simulink model "Piccolo_Induction_Motor"  (R2022b)
settings: Solver=FixedStepAuto  StartTime=0.0  StopTime=Inf  RelTol=1e-3  EnableMultiTasking=on
PostLoadFcn:
  | ,try, rti_mdl_postloadfcn(bdroot, 'UpdateModel', 320, 'rti1104'); catch, disp(lasterr); end,
undefined symbols (not defined in the file or in its folder): Km
libraries: Piccolo_Library x4, c2802xlib x1
settings Model: ExtModeTrigDuration=8  Creator=sb35user  LastModifiedBy=carls
settings SolverCC: ZeroCrossAlgorithm=Non-adaptive  AlgebraicLoopSolver=TrustRegion  AutoInsertRateTranBlk=on
settings DataIOCC: LimitDataPoints=on  SaveFormat=Array  SignalLoggingSaveFormat=ModelDataLogs  ReturnWorkspaceOutputs=off
settings OptimizationCC: BlockReduction=off  DefaultUnderspecifiedDataType=single  EnhancedBackFolding=on  PassReuseOutputArgsAs=Individual arguments  ExpressionDepthLimit=2147483647  InitFltsAndDblsToZero=on  MaxStackSize=1024  OptimizeBlockOrder=speed  DifferentSizesBufferReuse=on  OptimizationCustomize=off  DenormalBehavior=FlushToZero  EfficientTunableParamExpr=on
settings DebuggingCC: UnderspecifiedInitializationDetection=Classic  MergeDetectMultiDrivingBlocksExec=none  SolverPrmCheckMsg=warning  ParameterTunabilityLossMsg=error  FcnCallInpInsideContextMsg=warning  UnconnectedInputMsg=warning  UnconnectedOutputMsg=warning  UnconnectedLineMsg=warning  StateNameClashWarn=warning  SFUnexpectedBacktrackingDiag=warning  SFNoUnconditionalDefaultTransitionDiag=warning  SFExecutionAtInitializationDiag=none  SFMachineParentedDataDiag=warning  ArithmeticOperatorsInVariantConditions=warning
settings HardwareCC: ProdBitPerChar=16  ProdBitPerInt=16  ProdBitPerPointer=32  ProdBitPerSizeT=32  ProdBitPerPtrDiffT=32  ProdLargestAtomicInteger=Integer  ProdLargestAtomicFloat=None  ProdWordSize=16  ProdLongLongMode=on  ProdHWDeviceType=Texas Instruments->C2000  TargetIntDivRoundTo=Zero  TargetEndianess=BigEndian
settings ModelReferenceCC: PropagateSignalLabelsOutOfModel=off
settings SFSimCC: MATLABDynamicMemAlloc=off
settings RTWCC: Description=Embedded Coder  SystemTargetFile=ert.tlc  HardwareBoard=TI Piccolo F28069M LaunchPad  TLCOptions=-aInlineSetEventsForThisBaseRateFcn=TLC_FALSE -aSuppressMultiTaskScheduler=TLC_FALSE -aRateBasedStepFcn=1  TemplateMakefile=ert_default_tmf  Toolchain=Texas Instruments Code Composer Studio (C2000)
settings CodeAppCC: ForceParamTrailComments=on  IgnoreCustomStorageClasses=off  OperatorAnnotations=on  SimulinkDataObjDesc=on  SFDataObjDesc=on  InsertBlockDesc=on
settings ERTTargetCC: CodeReplacementLibrary=TI C28x  SupportContinuousTime=on  ExtModeTransport=4  ExtModeStaticAlloc=on  ExtModeAutomaticAllocSize=off  ExtModeMexFile=ext_xcp  ExtModeIntrfLevel=Level2 - Open
settings ConfigComp: CovMetricSettings=dw  CovSaveCumulativeToWorkspaceVar=on  CovSaveSingleToWorkspaceVar=on

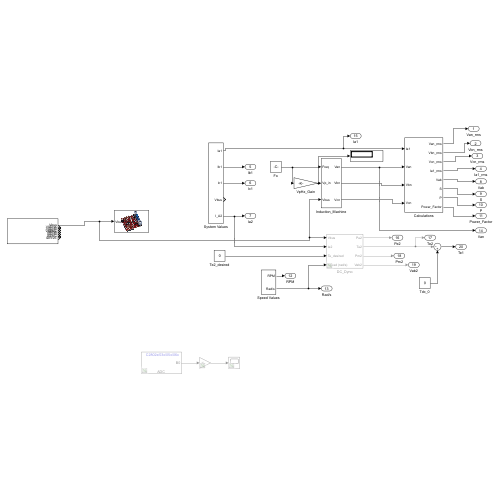
[thumbnail: Simulink's stored preview of the top-level diagram]
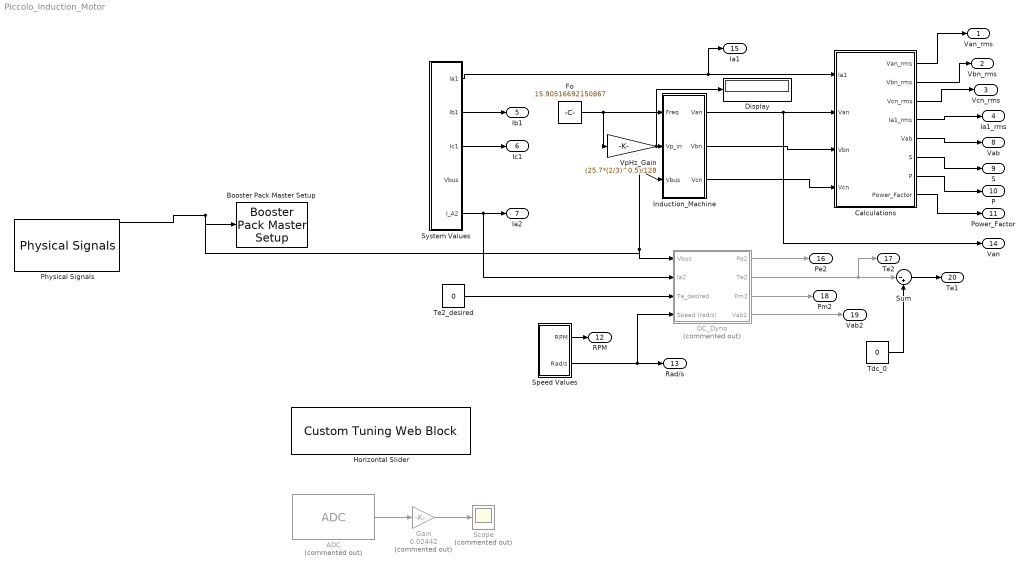
== system Piccolo_Induction_Motor ==
  ADC : c2802xlib/ADC  Commented=on  blkParamProc=C2000  ADCModule=1  samplingMode=Single sample mode  ADCResolution=12-bit (Single-ended input)  useSOC1=SOC0  useSOC2=SOC0_SOC1  SOCAcquisitionWindow=8  SOCTriggerSource=Software  SOCInterruptTrigger=No ADCINT  Ts=50e-6  dType=uint16  postInterrupt=off  interruptSel=ADCINT1  ADCINTContinuous=off  endma=off  chdma=1  conv1=ADCINB0  conv2=ADCINA0 and ADCINB0  conv1_Type4=ADCIN0  conv2_Type4=ADCIN0 and ADCIN1
      settings: LibrarySourceBlock=c2806xlib/ADC
  Booster Pack Master Setup : Piccolo_Library/Booster Pack Master Setup  SystemSampleTime=-1  VariantActivationTime=update diagram  Latency=0  AutoFrameSizeCalculation=off
      settings: SourceProductName=Piccolo Motor Control
  Calculations : Subsystem
  DC_Dyno : Subsystem  Commented=on
  Display : Display
  Fo : Constant  Value=15.90516692150867
  Gain : Gain  Commented=on  Gain=0.02442
  Horizontal Slider : CustomTuningWebBlock  LabelPosition=Hide  ShowInitialText=on  Configuration="{\"components\":[{\"name\":\"LinearScaleComponent\",\"settings\":{\"bounds\":{\"max\":60,\"min\":10,\"tickInterval\":\"auto\"},\"internalTickHeightScaleFactor\":0.5,\"labelColor\":[255,255,200],\"labelFont\":{\"font\":\"Arial\",\"fontSize\":12},\"labelOffset\":0.05,\"labelTransparency\":1,\"needleImage\":{\"size\":[596,842],\"src\":\"data:image\\/svg+xml;base64,PD94bWwgdmVyc2lvbj0iMS4wIiBlbmNvZGluZz0idXRmLTgiPz4NCjwhLS0gR2VuZXJhdG9yOiBBZG9iZSBJbGx1c3RyYXRvciAyNS4wLjAsIFNWRyBFeHBvcnQgUGx1Zy1JbiAuIFNWRyBWZXJzaW9uOiA2LjAwIEJ1aWxkIDApICAtLT4NCjxzdmcgdmVyc2lvbj0iMS4xIg0KCSBpZD0ic3ZnOCIgeG1sbnM6Y2M9Imh0dHA6Ly9jcmVhdGl2ZWNvbW1vbnMub3JnL25zIyIgeG1sbnM6ZGM9Imh0dHA6Ly9wdXJsLm9yZy9kYy9lbGVtZW50cy8xLjEvIiB4bWxuczppbmtzY2FwZT0iaHR0cDovL3d3dy5pbmtzY2FwZS5vcmcvbmFtZXNw ...(+2420 chars)\",\"srcOrientation\":\"Right\"},\"needleOffset\":[-0.8044596912521441,-0.0642123287671233],\"needleSize\":{\"height\":0.4337797619047619,\"width\":0.07668067226890757},\"position\":[0.2829861111111111,0.04398634453781513,0.9196428571428571,0.6088789682539683],\"referencePoint\":\"auto\",\"scaleColors\":[],\"scaleColorsSize\":0.2,\"scaleDirection\":\"LR\",\"showLabels\":1,\"showMinorTicks\":0,\"showSpanLine\":1,\"showTicks\":1,\"tickColor\":[252,252,197],\"tickTransparency\":1,\"valueBarColor\":[0,114,189],\"valueBarOffset\":-0.27,\"valueBarSize\":0.1,\"valueBarTransparency\":1}},{\"name\":\"BackgroundImageComponent\",\"settings\":{\"image\":{\"size\":[380,101],\"src\":\"data:image\\/svg+xml;base64,PHN2ZyB4bWxucz0iaHR0cDovL3d3dy53My5vcmcvMjAwMC9zdmciIHhtbG5zOnhsaW5rPSJodHRwOi8vd3d3LnczLm9yZy8xOTk5L3hsaW5rIiB2aWV3Qm94PSIwIDAgMzgwIDEwMSI+PGRlZnM+PHN0eWxlPi5jbHMtMXtmaWxsOiMwMDJiNDI7fS5jbHMtMntmaWxsOiM0MjcwODI7fS5jbHMtM3tmaWxsOnVybCgjcmFkaWFsLWdyYWRpZW50KTt9LmNscy00e2ZpbGw6I2M4YzhjODtzdHJva2U6IzAwMDt9PC9zdHlsZT48cmFkaWFsR3JhZGllbnQgaWQ9InJhZGlhbC1ncmFkaWVudCIgY3g9IjE5MCIgY3k9IjUwLjUiIHI9IjI2OS4yMSIgZ3JhZGllbnRVbml0cz0idXNlclNwYWNlT25Vc2UiPjxzdG9wIG9mZnNldD0iMC4wMSIgc3RvcC1jb2xvcj0iIzNlNGY1OCIvPjxzdG9wIG9mZnNldD0iMC4wNiIgc3RvcC1jb2xvcj0iIzQ0NTc2MSIvPjxzdG9wIG9mZnNldD0iMC4xNSIgc3RvcC1jb2xvcj0iIzU1NmE3NiIvPjxzdG9wIG9mZnNldD0iMC4yNSIgc3RvcC1jb2xvcj0iIzZkODg5NSIvPjxzdG9wIG9mZnNldD0iMC4zOCIgc3RvcC1jb2xvcj0iIzhmYjJjMyIvPjxzdG9wIG9mZnNldD0iMC41MiIgc3RvcC1jb2xvcj0iI2I2ZTRmYSIvPjxzdG9wIG9mZnNldD0iMSIgc3RvcC1jb2xvcj0iIzE1NDY1NyIvPjwvcmFkaWFsR3JhZGllbnQ+PC9kZWZzPjxnIGlkPSJmcmFtZSI+PGcgaWQ9IkxheWVyXzIiIGRhdGEtbmFtZT0iTGF5ZXIgMiI+PGcgaWQ9IkxheWVyXzEtMiIgZGF0YS1uYW1lPSJMYXllciAxLTIiPjxyZWN0IGlkPSJyZWN0MTAzNiIgY2xhc3M9ImNscy0xIiB4PSIxMSIgeT0iMTEiIHdpZHRoPSIzNTgiIGhlaWdodD0iNzkiLz48cGF0aCBpZD0icGF0aDEwMzgiIGNsYXNzPSJjbHMtMiIgZD0iTTgsOFY5M0gzNzJWOFpNMzY5LDkwSDExVjExSDM2OVoiLz48cGF0aCBpZD0icGF0aDEwNDAiIGNsYXNzPSJjbHMtMyIgZD0iTTAsMFYxMDFIMzgwVjBaTTM3Miw5M0g4VjhIMzcyWiIvPjwvZz48L2c+PC9nPjxnIGlkPSJ0cmFjayI+PHBhdGggaWQ9InJlY3QxNjExIiBjbGFzcz0iY2xzLTQiIGQ9Ik0zMy4zNywyNi41OUgzNDYuNjNjNCwwLDcuMjUsMi42LDcuMjUsNS44MWgwYzAsMy4yMS0zLjI1LDUuODItNy4yNSw1LjgySDMzLjM3Yy00LDAtNy4yNS0yLjYxLTcuMjUtNS44MmgwQzI2LjEyLDI5LjE5LDI5LjM3LDI2LjU5LDMzLjM3LDI2LjU5WiIvPjwvZz48L3N2Zz4=\",\"srcOrientation\":\"horizontal\"},\"position\":[0,0,1,1],\"scaleMode\":\"0\"}},{\"name\":\"ForegroundImageComponent\",\"settings\":{\"image\":{\"size\":[0,0],\"src\":\"default\",\"srcOrientation\":[]},\"isForeground\":1,\"position\":[0,0,1,1],\"scaleMode\":\"0\"}}],\"settings\":{\"BindingType\":\"param\",\"aspectRatio\":3.7777777777777777,\"backgroundColor\":[0,0,0,\"1\"],\"backgroundOffset\":0,\"backgroundOpacity\":1,\"fixedAspectRatio\":\"on\",\"foregroundColor\":[252,252,196],\"orientation\":\"horizontal\",\"showBackgroundColor\":false,\"value\":0,\"version\":\"R2022b\"},\"type\":\"LinearGauge\"}"
  Induction_Machine : Subsystem
  Physical Signals : Piccolo_Library/Physical Signals  Pack=1
      settings: SourceProductName=Piccolo Motor Control
  Scope : Scope  Commented=on
  Speed Values : Subsystem
  Sum : Sum  Inputs=|-+
  System Values : Subsystem
  Tdc_0 : Constant  Value=0
  Te2_desired : Constant  Value=0
  VpHz_Gain : Gain  Gain=(25.7*(2/3)^0.5)/128
  Van_rms : Outport
  Vbn_rms : Outport  Port=2
  Vcn_rms : Outport  Port=3
  Ia1_rms : Outport  Port=4
  Ib1 : Outport  Port=5
  Ic1 : Outport  Port=6
  Ia2 : Outport  Port=7
  Vab : Outport  Port=8
  S : Outport  Port=9
  P : Outport  Port=10
  Power_Factor : Outport  Port=11
  RPM : Outport  Port=12
  Rad/s : Outport  Port=13
  Van : Outport  Port=14
  Ia1 : Outport  Port=15
  Pe2 : Outport  Port=16
  Te2 : Outport  Port=17
  Pm2 : Outport  Port=18
  Vab2 : Outport  Port=19
  Te1 : Outport  Port=20
  wires:
  System Values/2(Ib1) -> Ib1/1
  System Values/3(Ic1) -> Ic1/1
  Fo/1 -> Induction_Machine/1(Freq), VpHz_Gain/1
  System Values/5(I_A2) -> Ia2/1, DC_Dyno/2(Ia2)
  Induction_Machine/3(Vcn) -> Calculations/4(Vcn)
  System Values/1(Ia1) -> Calculations/1(Ia1), Ia1/1
  Induction_Machine/1(Van) -> Calculations/2(Van), Van/1
  Induction_Machine/2(Vbn) -> Calculations/3(Vbn)
  Calculations/1(Van_rms) -> Van_rms/1
  Calculations/2(Vbn_rms) -> Vbn_rms/1
  Calculations/3(Vcn_rms) -> Vcn_rms/1
  Calculations/4(Ia1_rms) -> Ia1_rms/1
  Calculations/5(Vab) -> Vab/1
  Calculations/6(S) -> S/1
  Calculations/7(P) -> P/1
  Calculations/8(Power_Factor) -> Power_Factor/1
  Speed Values/1(RPM) -> RPM/1
  Speed Values/2(Rad/s) -> Rad/s/1, DC_Dyno/4(Speed (rad/s))
  Te2_desired/1 -> DC_Dyno/3(Te_desired)
  DC_Dyno/1(Pe2) -> Pe2/1
  DC_Dyno/3(Pm2) -> Pm2/1
  DC_Dyno/4(Vab2) -> Vab2/1
  DC_Dyno/2(Te2) -> Sum/1, Te2/1
  Tdc_0/1 -> Sum/2
  Sum/1 -> Te1/1
  Physical Signals/1 -> Induction_Machine/3(Vbus), DC_Dyno/1(Vbus), Booster Pack Master Setup/1
  Gain/1 -> Scope/1
  ADC/1 -> Gain/1
  VpHz_Gain/1 -> Display/1, Induction_Machine/2(Vp_in)

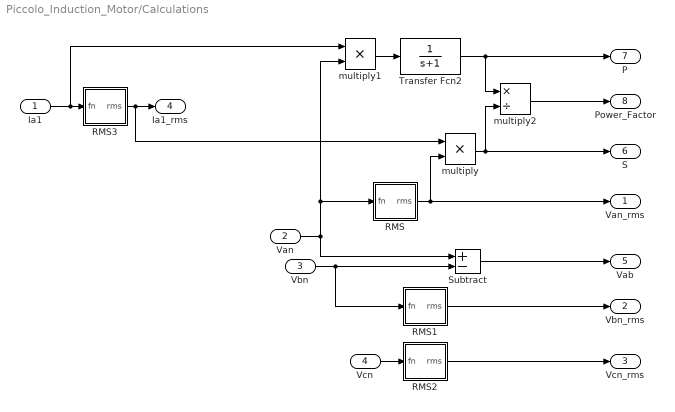
== system Piccolo_Induction_Motor/Calculations ==
  Ia1 : Inport
  Van : Inport  Port=2
  Vbn : Inport  Port=3
  Vcn : Inport  Port=4
  RMS : Subsystem
  RMS1 : Subsystem
  RMS2 : Subsystem
  RMS3 : Subsystem
  Subtract : Sum  Inputs=+-
  Transfer Fcn2 : TransferFcn  Denominator=[1 1]
  multiply : Product  Inputs=**
  multiply1 : Product  Inputs=**
  multiply2 : Product  Inputs=*/
  Van_rms : Outport
  Vbn_rms : Outport  Port=2
  Vcn_rms : Outport  Port=3
  Ia1_rms : Outport  Port=4
  Vab : Outport  Port=5
  S : Outport  Port=6
  P : Outport  Port=7
  Power_Factor : Outport  Port=8
  wires:
  Subtract/1 -> Vab/1
  Van/1 -> multiply1/2, RMS/1(fn), Subtract/1
  Vbn/1 -> RMS1/1(fn), Subtract/2
  RMS/1(rms) -> Van_rms/1, multiply/2
  RMS1/1(rms) -> Vbn_rms/1
  RMS2/1(rms) -> Vcn_rms/1
  Ia1/1 -> multiply1/1, RMS3/1(fn)
  RMS3/1(rms) -> Ia1_rms/1, multiply/1
  multiply/1 -> S/1, multiply2/2
  Transfer Fcn2/1 -> P/1, multiply2/1
  multiply1/1 -> Transfer Fcn2/1
  multiply2/1 -> Power_Factor/1
  Vcn/1 -> RMS2/1(fn)

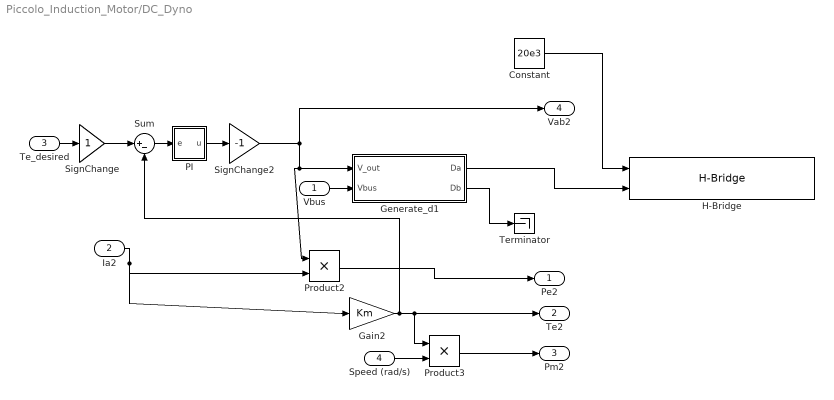
== system Piccolo_Induction_Motor/DC_Dyno ==
  Vbus : Inport
  Ia2 : Inport  Port=2
  Te_desired : Inport  Port=3
  Speed (rad/s) : Inport  Port=4
  Constant : Constant  Value=20e3
  Gain2 : Gain  Gain=Km
  Generate_d1 : Subsystem
  H-Bridge : Piccolo_Library/H-Bridge  Pack=1  Prescale=8
      settings: SourceProductName=Piccolo Motor Control
  PI : Subsystem
  Product2 : Product  RndMeth=Zero
  Product3 : Product  RndMeth=Zero
  SignChange : Gain
  SignChange2 : Gain  Gain=-1
  Sum : Sum  Inputs=|+-
  Terminator : Terminator
  Pe2 : Outport
  Te2 : Outport  Port=2
  Pm2 : Outport  Port=3
  Vab2 : Outport  Port=4
  wires:
  PI/1(u) -> SignChange2/1
  Generate_d1/1(Da) -> H-Bridge/2
  Generate_d1/2(Db) -> Terminator/1
  Product2/1 -> Pe2/1
  Product3/1 -> Pm2/1
  Sum/1 -> PI/1(e)
  Gain2/1 -> Sum/2, Te2/1, Product3/1
  Vbus/1 -> Generate_d1/2(Vbus)
  Ia2/1 -> Product2/2, Gain2/1
  Speed (rad/s)/1 -> Product3/2
  Te_desired/1 -> SignChange/1
  SignChange/1 -> Sum/1
  SignChange2/1 -> Product2/1, Generate_d1/1(V_out), Vab2/1
  Constant/1 -> H-Bridge/1

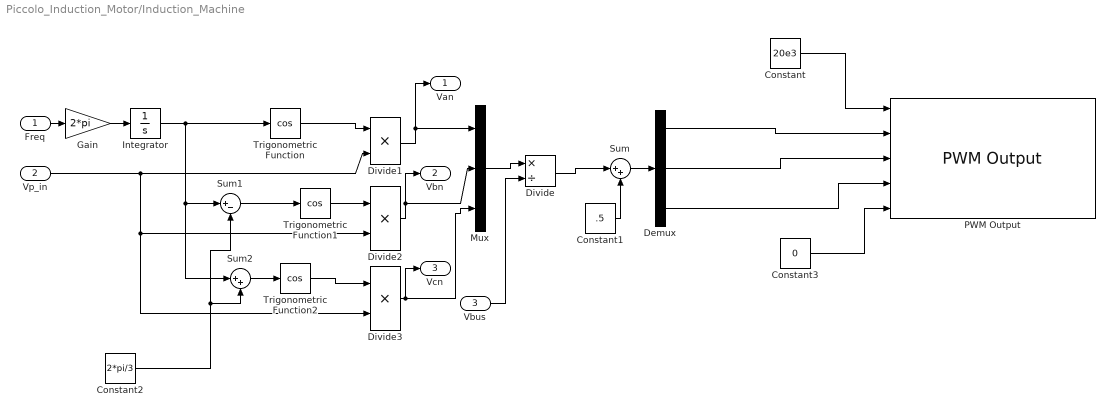
== system Piccolo_Induction_Motor/Induction_Machine ==
  Freq : Inport
  Vp_in : Inport  Port=2
  Vbus : Inport  Port=3
  Constant : Constant  Value=20e3
  Constant1 : Constant  Value=.5
  Constant2 : Constant  Value=2*pi/3
  Constant3 : Constant  Value=0
  Demux : Demux  Outputs=3
  Divide : Product  Inputs=*/
  Divide1 : Product  Inputs=**
  Divide2 : Product  Inputs=**
  Divide3 : Product  Inputs=**
  Gain : Gain  Gain=2*pi
  Integrator : Integrator
  Mux : Mux  Inputs=3
  PWM Output : Piccolo_Library/PWM Output  Pack=1  Prescale=1
      settings: SourceProductName=Piccolo Motor Control
  Sum : Sum  Inputs=|++
  Sum1 : Sum  Inputs=|+-
  Sum2 : Sum  Inputs=|++
  Trigonometric Function : Trigonometry  Operator=cos
  Trigonometric Function1 : Trigonometry  Operator=cos
  Trigonometric Function2 : Trigonometry  Operator=cos
  Van : Outport
  Vbn : Outport  Port=2
  Vcn : Outport  Port=3
  wires:
  Constant1/1 -> Sum/2
  Sum/1 -> Demux/1
  Mux/1 -> Divide/1
  Divide/1 -> Sum/1
  Vbus/1 -> Divide/2
  Gain/1 -> Integrator/1
  Freq/1 -> Gain/1
  Integrator/1 -> Trigonometric Function/1, Sum2/1, Sum1/1
  Trigonometric Function/1 -> Divide1/1
  Vp_in/1 -> Divide1/2, Divide2/2, Divide3/2
  Divide1/1 -> Mux/1, Van/1
  Sum1/1 -> Trigonometric Function1/1
  Divide2/1 -> Mux/2, Vbn/1
  Trigonometric Function1/1 -> Divide2/1
  Constant2/1 -> Sum1/2, Sum2/2
  Sum2/1 -> Trigonometric Function2/1
  Trigonometric Function2/1 -> Divide3/1
  Divide3/1 -> Mux/3, Vcn/1
  Demux/1 -> PWM Output/2
  Demux/2 -> PWM Output/3
  Demux/3 -> PWM Output/4
  Constant/1 -> PWM Output/1
  Constant3/1 -> PWM Output/5

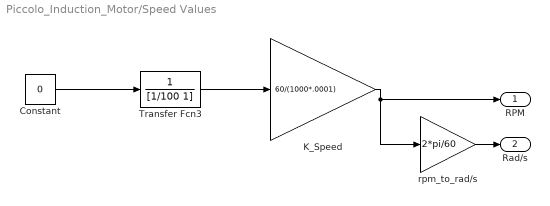
== system Piccolo_Induction_Motor/Speed Values ==
  Constant : Constant  Value=0
  K_Speed : Gain  Gain=60/(1000*.0001)
  Transfer Fcn3 : TransferFcn  Denominator=[1/100 1]
  rpm_to_rad/s : Gain  Gain=2*pi/60
  RPM : Outport
  Rad/s : Outport  Port=2
  wires:
  K_Speed/1 -> rpm_to_rad/s/1, RPM/1
  rpm_to_rad/s/1 -> Rad/s/1
  Constant/1 -> Transfer Fcn3/1
  Transfer Fcn3/1 -> K_Speed/1

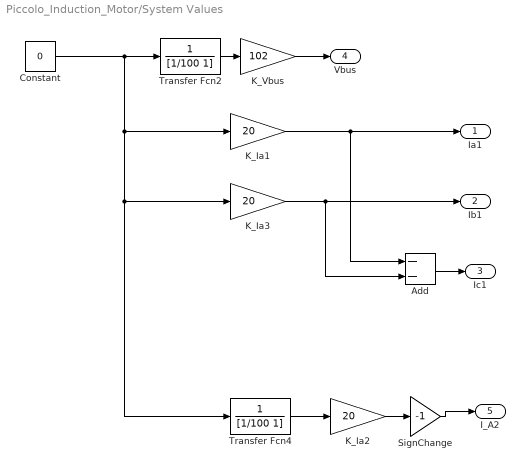
== system Piccolo_Induction_Motor/System Values ==
  Add : Sum  Inputs=--
  Constant : Constant  Value=0
  K_Ia1 : Gain  Gain=20
  K_Ia2 : Gain  Gain=20
  K_Ia3 : Gain  Gain=20
  K_Vbus : Gain  Gain=102
  SignChange : Gain  Gain=-1
  Transfer Fcn2 : TransferFcn  Denominator=[1/100 1]
  Transfer Fcn4 : TransferFcn  Denominator=[1/100 1]
  Ia1 : Outport
  Ib1 : Outport  Port=2
  Ic1 : Outport  Port=3
  Vbus : Outport  Port=4
  I_A2 : Outport  Port=5
  wires:
  Transfer Fcn4/1 -> K_Ia2/1
  Constant/1 -> Transfer Fcn4/1, K_Ia3/1, K_Ia1/1, Transfer Fcn2/1
  K_Ia2/1 -> SignChange/1
  Transfer Fcn2/1 -> K_Vbus/1
  K_Ia1/1 -> Ia1/1, Add/1
  K_Vbus/1 -> Vbus/1
  K_Ia3/1 -> Ib1/1, Add/2
  Add/1 -> Ic1/1
  SignChange/1 -> I_A2/1

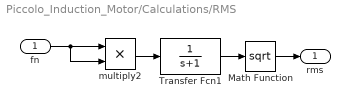
== system Piccolo_Induction_Motor/Calculations/RMS ==
  fn : Inport
  Math Function : Math  Operator=sqrt  SignedPower=on
  Transfer Fcn1 : TransferFcn  Denominator=[1 1]
  multiply2 : Product  Inputs=**
  rms : Outport
  wires:
  multiply2/1 -> Transfer Fcn1/1
  Transfer Fcn1/1 -> Math Function/1
  fn/1 -> multiply2/1, multiply2/2
  Math Function/1 -> rms/1

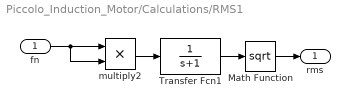
== system Piccolo_Induction_Motor/Calculations/RMS1 ==
  fn : Inport
  Math Function : Math  Operator=sqrt  SignedPower=on
  Transfer Fcn1 : TransferFcn  Denominator=[1 1]
  multiply2 : Product  Inputs=**
  rms : Outport
  wires:
  Math Function/1 -> rms/1
  fn/1 -> multiply2/2, multiply2/1
  Transfer Fcn1/1 -> Math Function/1
  multiply2/1 -> Transfer Fcn1/1

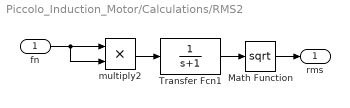
== system Piccolo_Induction_Motor/Calculations/RMS2 ==
  fn : Inport
  Math Function : Math  Operator=sqrt  SignedPower=on
  Transfer Fcn1 : TransferFcn  Denominator=[1 1]
  multiply2 : Product  Inputs=**
  rms : Outport
  wires:
  multiply2/1 -> Transfer Fcn1/1
  Transfer Fcn1/1 -> Math Function/1
  fn/1 -> multiply2/1, multiply2/2
  Math Function/1 -> rms/1

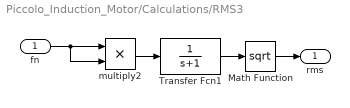
== system Piccolo_Induction_Motor/Calculations/RMS3 ==
  fn : Inport
  Math Function : Math  Operator=sqrt  SignedPower=on
  Transfer Fcn1 : TransferFcn  Denominator=[1 1]
  multiply2 : Product  Inputs=**
  rms : Outport
  wires:
  Math Function/1 -> rms/1
  fn/1 -> multiply2/2, multiply2/1
  Transfer Fcn1/1 -> Math Function/1
  multiply2/1 -> Transfer Fcn1/1

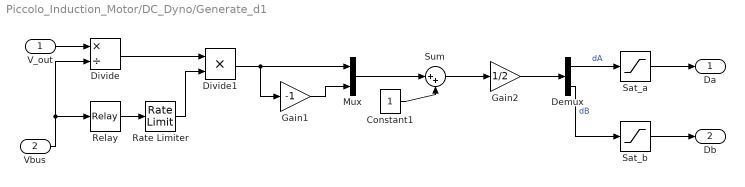
== system Piccolo_Induction_Motor/DC_Dyno/Generate_d1 ==
  V_out : Inport
  Vbus : Inport  Port=2
  Constant1 : Constant
  Demux : Demux  Outputs=2
  Divide : Product  Inputs=*/
  Divide1 : Product  Inputs=**
  Gain1 : Gain  Gain=-1
  Gain2 : Gain  Gain=1/2
  Mux : Mux  Inputs=2
  Rate Limiter : RateLimiter  RisingSlewLimit=.7  SampleTimeMode=inherited
  Relay : Relay  OnSwitchValue=10  OffSwitchValue=10
  Sat_a : Saturate  UpperLimit=.98  LowerLimit=0
  Sat_b : Saturate  UpperLimit=.98  LowerLimit=0
  Sum : Sum  Inputs=|++
  Da : Outport
  Db : Outport  Port=2
  wires:
  Divide1/1 -> Gain1/1, Mux/1
  Rate Limiter/1 -> Divide1/2
  Divide/1 -> Divide1/1
  Relay/1 -> Rate Limiter/1
  Sat_b/1 -> Db/1
  Sat_a/1 -> Da/1
  Demux/2 -> Sat_b/1  "dB"
  Vbus/1 -> Relay/1, Divide/2
  Demux/1 -> Sat_a/1  "dA"
  V_out/1 -> Divide/1
  Gain2/1 -> Demux/1
  Sum/1 -> Gain2/1
  Gain1/1 -> Mux/2
  Mux/1 -> Sum/1
  Constant1/1 -> Sum/2

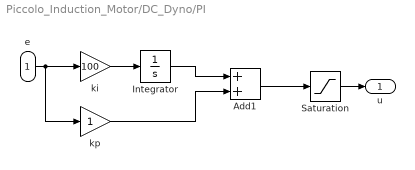
== system Piccolo_Induction_Motor/DC_Dyno/PI ==
  e : Inport
  Add1 : Sum
  Integrator : Integrator  LimitOutput=on  UpperSaturationLimit=42  LowerSaturationLimit=-42
  Saturation : Saturate  UpperLimit=42  LowerLimit=-42
  ki : Gain  Gain=100
  kp : Gain
  u : Outport
  wires:
  e/1 -> kp/1, ki/1
  Add1/1 -> Saturation/1
  kp/1 -> Add1/2
  Integrator/1 -> Add1/1
  ki/1 -> Integrator/1
  Saturation/1 -> u/1
